simulink model "MPC"  (R2017a)
settings: Solver=VariableStepAuto  StartTime=0.0  StopTime=10.0  RelTol=1e-3
values from neighbouring files (symbols this model uses):
  I1 = 1.17    [sistemacontrolado.m]
  I2 = 3    [sistemacontrolado.m]
  R = Ra1    (= 28.8)    [sistemacontrolado.m]
libraries: powerlib x7, instrumentlib x4, mpclib x1
settings Model: Creator=MarioAndres  LastModifiedBy=MarioAndres

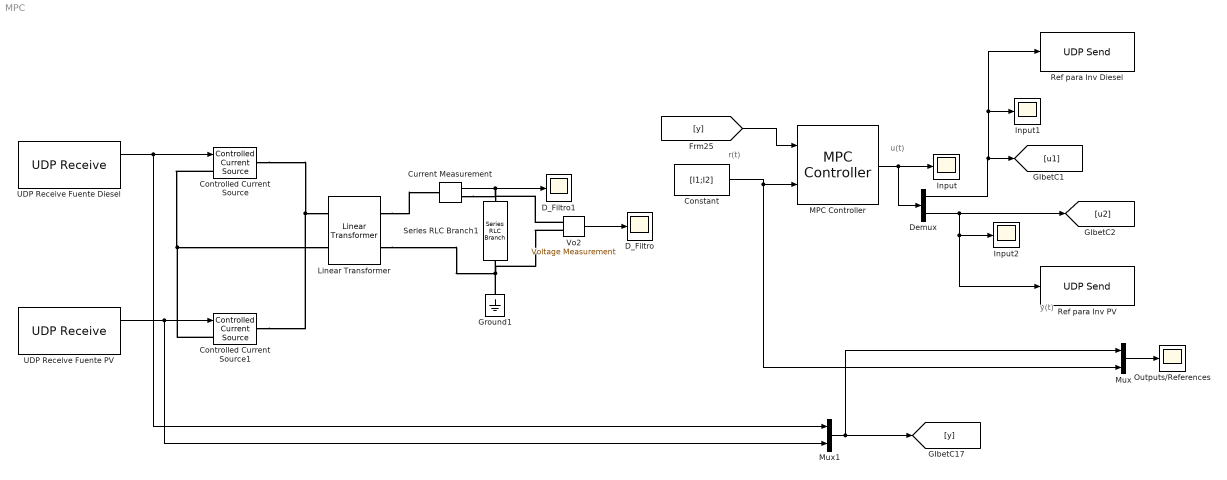
== system MPC ==
  note: u(t)
  note: y(t)
  note: r(t)
  Constant : Constant  Value=[I1;I2]
  Controlled Current Source : powerlib/Electrical Sources/Controlled Current Source  Initialize=on  Source_Type=AC  Amplitude=0  Phase=0  Frequency=0  Measurements=None
  Controlled Current Source1 : powerlib/Electrical Sources/Controlled Current Source  Initialize=on  Source_Type=AC  Amplitude=0  Phase=0  Frequency=0  Measurements=None
  Current Measurement : powerlib/Measurements/Current Measurement  PhasorSimulation=off  OutputType=Complex  PSBequivalent=0
  D_Filtro : Scope
  D_Filtro1 : Scope
  Demux : Demux  Outputs=2
  Ground1 : powerlib/Elements/Ground  LConnTagsString=a
  Input : Scope
  Input1 : Scope
  Input2 : Scope
  Linear Transformer : powerlib/Elements/Linear Transformer  UNITS=SI  NominalPower=[ 1500 60 ]  winding1=[141.2 0 0.003]  winding2=[120 0.004 0.084225]  ThreeWindings=off  winding3=[3.15e+05 0.7938 0.084225]  RmLm=[1.0805e+06 2866]  Measurements=None  DataType=on
  MPC Controller : mpclib/MPC Controller  mpcobj=mpcobj  x0=[]  is_multiple=0  enable_value=0  return_u0=off  ref_from_ws=off  ref_signal_name=[]  ref_preview=on  md_from_ws=off  md_signal_name=[]  md_preview=on  from_project=off  project_file=MPCtask.mat  md_inport=off  mv_inport=off  cost_outport=off  return_sequence=off  return_qpstatus=off  return_state=off  state_inport=off  lims_inport=off  ywt_inport=off  is_designfromscratch=0  uwt_inport=off  duwt_inport=off  rhoeps_inport=off  uref_inport=off  n_ts=0.1  n_mv=2  n_md=0  n_ud=0  n_mo=2  n_uo=0  BlockDataType=double  SampleTimeInherited=off  switch_inport=off
  Mux : Mux  Inputs=2
  Mux1 : Mux  Inputs=2
  Outputs/References : Scope
  Ref para Inv Diesel : instrumentlib/UDP Send  Priority=2  Host=169.254.26.197  Port=51006  LocalPort=51007  EnableBlockingMode=on  ByteOrder=BigEndian
      settings: SourceProductName=Instrument Control Toolbox
  Ref para Inv PV : instrumentlib/UDP Send  Priority=2  Host=196.254.26.15  Port=51002  LocalPort=51003  EnableBlockingMode=on  ByteOrder=BigEndian
      settings: SourceProductName=Instrument Control Toolbox
  Series RLC Branch1 : powerlib/Elements/Series RLC Branch  LConnTagsString=__new0  RConnTagsString=__new0  BranchType=R  Resistance=R  Inductance=25e-3  SetiL0=off  InitialCurrent=0  Capacitance=5.30e-3  Setx0=off  InitialVoltage=0  Measurements=None
  UDP Receive Fuente Diesel : instrumentlib/UDP Receive  Host=169.254.26.197  Port=51006  LocalPort=51007  DataSize="[6  1]"  EnableBlockingMode=off  Timeout=1  SampleTime=1  DataType=uint8  ByteOrder=BigEndian
      settings: SourceProductName=Instrument Control Toolbox
  UDP Receive Fuente PV : instrumentlib/UDP Receive  Host=169.254.26.15  Port=51002  LocalPort=51003  DataSize="[6  1]"  EnableBlockingMode=off  Timeout=1  SampleTime=1  DataType=uint8  ByteOrder=BigEndian
      settings: SourceProductName=Instrument Control Toolbox
  Vo2 : powerlib/Measurements/Voltage Measurement  PhasorSimulation=off  OutputType=Complex  PSBequivalent=0
  wires:
  [y] -> MPC Controller/1
  Demux/2 -> Ref para Inv PV/1, Input2/1, [u2]
  Constant/1 -> Mux/2, MPC Controller/2
  Mux/1 -> Outputs/References/1
  MPC Controller/1 -> Demux/1, Input/1
  Demux/1 -> Ref para Inv Diesel/1, Input1/1, [u1]
  Vo2/1 -> D_Filtro/1
  Current Measurement/1 -> D_Filtro1/1
  UDP Receive Fuente PV/1 -> Mux1/2, Controlled Current Source1/1
  Mux1/1 -> Mux/1, [y]
  UDP Receive Fuente Diesel/1 -> Mux1/1, Controlled Current Source/1
  connections:
  Series RLC Branch1/LConn1 -- Vo2/LConn1 -- Current Measurement/RConn1
  Series RLC Branch1/RConn1 -- Ground1/LConn1 -- Linear Transformer/RConn2 -- Vo2/LConn2
  Linear Transformer/RConn1 -- Current Measurement/LConn1
  Controlled Current Source/RConn1 -- Controlled Current Source1/RConn1 -- Linear Transformer/LConn1
  Controlled Current Source/LConn1 -- Controlled Current Source1/LConn1 -- Linear Transformer/LConn2
